simulink model "NewDiscrete"  (R2019b)
settings: Solver=VariableStepAuto  StartTime=0.0  StopTime=10.0  RelTol=1e-3
settings Model: Creator=trulsmartinsson  LastModifiedBy=trulsmartinsson

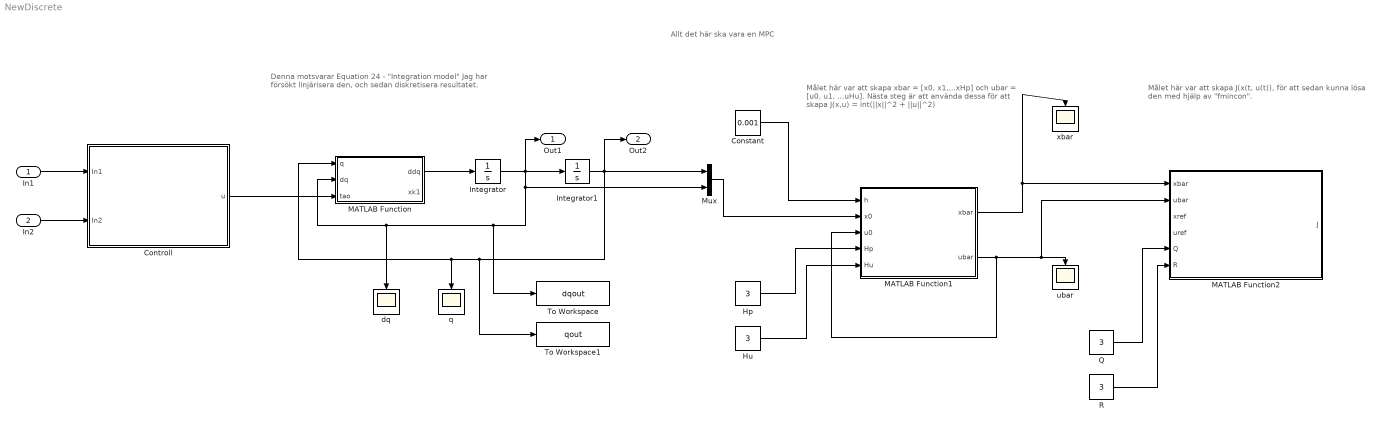
== system NewDiscrete ==
  note: Allt det här ska vara en MPC
  note: Målet här var att skapa J(x(t, u(t)), för att sedan
      | kunna lösa den med hjälp av "fmincon".
  note: Målet här var att skapa xbar = [x0, x1,...xHp]
      | och ubar = [u0, u1, ...uHu].
      | Nästa steg är att använda dessa för att skapa
      | J(x,u) = int(||x||^2 + ||u||^2)
  note: Denna motsvarar
      | Equation 24 - "Integration model"
      | Jag har försökt linjärisera den, och sedan
      | diskretisera resultatet.
  In1 : Inport
  In2 : Inport  Port=2
  Constant : Constant  Value=0.001
  Controll : Subsystem
  "Hp " : Constant  Value=3
  "Hu " : Constant  Value=3
  Integrator : Integrator  InitialCondition=[0;pi/6]
  Integrator1 : Integrator  InitialCondition=[0;0]
  MATLAB Function : MATLAB Function  TreatAsAtomicUnit=on
  MATLAB Function1 : MATLAB Function  TreatAsAtomicUnit=on
  MATLAB Function2 : MATLAB Function  TreatAsAtomicUnit=on
  Mux : Mux  Inputs=2
  Q : Constant  Value=3
  R : Constant  Value=3
  To Workspace : ToWorkspace  VariableName=dqout  SaveFormat=Timeseries  SampleTime=-1
  To Workspace1 : ToWorkspace  VariableName=qout  SampleTime=-1
  dq : Scope
  q : Scope
  ubar : Scope
  xbar : Scope
  Out1 : Outport
  Out2 : Outport  Port=2
  wires:
  Integrator/1 -> Mux/2, To Workspace/1, dq/1, MATLAB Function/2(dq), Integrator1/1, Out1/1
  Integrator1/1 -> Mux/1, To Workspace1/1, MATLAB Function/1(q), q/1, Out2/1
  MATLAB Function/1(ddq) -> Integrator/1
  In1/1 -> Controll/1(In1)
  In2/1 -> Controll/2(In2)
  Controll/1(u) -> MATLAB Function/3(tao)
  Constant/1 -> MATLAB Function1/1(h)
  "Hp "/1 -> MATLAB Function1/4(Hp)
  "Hu "/1 -> MATLAB Function1/5(Hu)
  MATLAB Function1/1(xbar) -> MATLAB Function2/1(xbar), xbar/1
  MATLAB Function1/2(ubar) -> MATLAB Function1/3(u0), MATLAB Function2/2(ubar), ubar/1
  Mux/1 -> MATLAB Function1/2(x0)
  Q/1 -> MATLAB Function2/5(Q)
  R/1 -> MATLAB Function2/6(R)

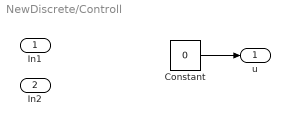
== system NewDiscrete/Controll ==
  In1 : Inport
  In2 : Inport  Port=2
  Constant : Constant  Value=0
  u : Outport
  wires:
  Constant/1 -> u/1

== matlab function NewDiscrete/MATLAB Function1 ==
  data: h input; x0 input; u0 input; xbar output [0..4*Hp]; ubar output; Hp input; Hu input
function [xbar, ubar] = createBars(h, x0, u0, Hp, Hu)
%Input vector xk = [phi_k, dphi_k, theta_k, dtheta_k], and time step h;
%Output vector xk1 = [phi_{k+1}, dphi_{k+1}, theta_{k+1}, dtheta_{k+1}];

%x = [phi, dphi, theta, dtheta]';    %This is the most recent x (x_k)

if (length(x0) < 4*Hp)
    xbar = zeros(4*Hp,1);
    xbar(1:4) = x0;
else
    xbar = x0;      
end

if (length(u0) < 2*Hu)
    ubar = zeros(2*Hu,1);
    ubar(1:2) = u0;
else
    ubar = u0;
end


%%

la  = 75*10^-3;       %[m]      - Length of arm
r  = 43*10^-3;       %[m]      - Base radius
lp  = 31.5*10^-3;     %[m]      - Length of pendulum
J  = 125*10^-6;      %[kgm^2]  - Base moment of inertia
g  = 9.8;            %[m/s^2]  - Gravity
Jc = 2.55*10^-6;     %[kgm^2]  - Moment of inertia of pendulum around c.o.m
M  = 5.44*10^-3;     %[kg]     - Mass of pendulum point mass
Jp = 7.95*10^-6;     %[kgm^2]  - Moment of inertia of pend around pivot

%Still unknown - Try to guess these as a first step
ma = 10*10^-3;       %[kg] - Mass of arm       - Try 10g
mp = 5*10^-3;        %[kg] - Mass of pendulum  - Try 5g

%Equation (17)
alpha   = J + (M + (1/3)*ma + mp)*la^2;
beta    = (M + (1/3)*mp)*lp^2;
gamma   = (M + (1/2)*mp)*la*lp;
delta   = (M + (1/2)*mp)*g*lp;
denum = alpha*beta - gamma^2;

A = [0 1 0 0;
    0 0 -delta*gamma/denum 0;
    0 0 0 1;
    0 0 -alpha*delta/denum 0];
B = [0 0;
    beta/denum -gamma/denum;
    0 0;
    -gamma/denum alpha/denum];
%%

Ahp = zeros(4*Hp,4*Hp);
Bhu = zeros(4*Hu,2*Hu);
for i = 1:Hp
    Ahp((4*i-3):(4*i), 1:4) = (1+h*A)^i;        %AHp stämmer nog
end
Brow = zeros(4, 2*Hu);
Brow(1:4, 1:2) = h*B;
Bhu(1:4,:) = Brow;
for j = 2:Hu
    Brow = circshift(Brow',2)';
    Brow(1:4,1:2) = (h*B'*(1+h*A)^(j-1))';
    Bhu(4*j-3:4*j, :) = Brow;
end

xk1 = Ahp(1:4,:)*xbar + Bhu(1:4,:)*ubar;
xbar(1:4,1) = x0(1:4);
xbar = circshift(xbar, 4);
xbar(1:4,1) = xk1(1:4)';
ubar(1:2, 1) = u0(1:2);
ubar = circshift(ubar,2);
%Hur ska ubar uppdateras?

end

== matlab function NewDiscrete/MATLAB Function ==
  data: q input; ddq output; dq input; tao input; xk1 output
function  [ddq, xk1] = discretized(q,dq,tao)
%Equation 30 - Linearized model -> Discrete
%% q= [phi, theta],   dq = [dphi, dtheta]
tao2=[0;tao];
%tao2 =[tao;1];
phi = q(1,1);
dphi = dq(1,1);
theta = q(2,1);
dtheta = dq(2,1);
x = [phi, dphi, theta, dtheta]';

%Given parameters - "competition.pdf"
la  = 75*10^-3;       %[m]      - Length of arm
r  = 43*10^-3;       %[m]      - Base radius
lp  = 31.5*10^-3;     %[m]      - Length of pendulum
J  = 125*10^-6;      %[kgm^2]  - Base moment of inertia
g  = 9.8;            %[m/s^2]  - Gravity
Jc = 2.55*10^-6;     %[kgm^2]  - Moment of inertia of pendulum around c.o.m
M  = 5.44*10^-3;     %[kg]     - Mass of pendulum point mass
Jp = 7.95*10^-6;     %[kgm^2]  - Moment of inertia of pend around pivot

%Still unknown - Try to guess these as a first step
ma = 10*10^-3;       %[kg] - Mass of arm       - Try 10g
mp = 5*10^-3;        %[kg] - Mass of pendulum  - Try 5g

%Equation (17)
alpha   = J + (M + (1/3)*ma + mp)*la^2;
beta    = (M + (1/3)*mp)*lp^2;
gamma   = (M + (1/2)*mp)*la*lp;
delta   = (M + (1/2)*mp)*g*lp;

denum = alpha*beta - gamma^2;
phi = q(1,1);

x = [phi, dphi, theta, dtheta]';
A = [0 1 0 0;
    0 0 -delta*gamma/denum 0;
    0 0 0 1;
    0 0 -alpha*delta/denum 0];
B = [0 0;
    beta/denum -gamma/denum;
    0 0;
    -gamma/denum alpha/denum];
C=[ 0,1,0,0;
    0,0,0,1];
D=[ 0,0;
    0,0];
dx = A*x + B*tao2;

% q 
% dq
ddq = C*dx + D*tao2

%Step 2: Discretize -> x_{k+1} = (1+hA)x_{k} + hBu_{k}
h = 0.001;          %time step in [s]
Ad = [1 1+h 1 1;
      1 1 (1 - (h*delta*gamma/denum)) 1;
      1 1 1 1+4;
      1 1 (1+ (h*alpha*delta/denum)) 1];
Bd = [0 0;
      beta/denum, -gamma/denum;
      0 0;
      -gamma/denum alpha/denum];
%Print out the discretized output, xk1 = [phi_{k+1}, phi_{k+2}, theta_{k+1}, theta_{k+2}]  
xk1 = Ad*x + h*Bd*tao2;





%\dot{x} = Ax + Bu -> x_{k+1} = (1+hA)x_{k} + hBu_{k}



% ddq = inv(D)*(tao2 - C*dq - G);
%ddq = D\(tao2 - C*dq - G);




%Truls testar att plocka ut q, dq som vektorer
% if(q(2) >= 22)
%     disp('q > 22, OVER!');
% else
%     disp('q < 22, UNDER!');
% end
end

== matlab function NewDiscrete/MATLAB Function2 ==
  data: xbar input; J output; ubar input; xref input; uref input; Q input; R input
function J  = formJacobian(xbar, ubar, xref, uref, Q, R)
%Try to form the Jacobian defined as J(x,u) = int{||x||^2 + ||u||^2}

%1) Skapa QORO
%2) Multiplicera [(xbar-xbar^r);(ubar-ubar^r))]'*QORO*[xbar-xbar^r] för att få ||x||^2
x = [xbar; ubar];
xr = [xref; uref];
Qmat = Q*eye(length(xbar));
Rmat = R*eye(length(ubar));
QORO = zeros(length(xbar)+length(ubar));
QORO(1:length(xbar),1:length(xbar)) = Qmat;
QORO(length(xbar)+1:end, length(xbar)+1:end) = Rmat;

J = (x-xr)'*QORO*(x-xr);

end
